simulink model "MatLab5"  (Simulink 8.7)
settings: Solver=ode45  StartTime=0.0  StopTime=100  MaxStep=0.01  RelTol=1e-3
values from neighbouring files (symbols this model uses):
  A = [0 1  0              0 ... (first row only)    [MatLab4p.m]    (also in MatLab5p.m = [     0        1       0        0; MatLab6p.m = [     0        1       0        0; _Labs.m = [     0        1       0        0; q2.m = [0 1  0   0)
  Am = blkdiag(M,M)    [MatLab5p.m]    (also in MatLab6p.m; _Labs.m; q2.m = 1; questao2.m = 1)
  B = [0; 1/M; 0; -1/(M*L)]    [MatLab4p.m]    (also in MatLab5p.m = [ 0    0; MatLab6p.m = [ 0    0; _Labs.m = [ 0    0; q2.m = [  0)
  Bm = blkdiag(N,N)    [MatLab5p.m]    (also in MatLab6p.m; _Labs.m; q2.m = N; questao2.m = N)
  C = [1 0 0 0]    [MatLab4p.m]    (also in MatLab5p.m = [1 0 0 0; MatLab6p.m = [1 0 0 0; _Labs.m = [1 0 0 0; q2.m)
  Dsim = zeros(4,1)    [MatLab4p.m]    (also in MatLab5p.m = zeros(4,2); MatLab6p.m = zeros(4,2); _Labs.m = zeros(4,2); q2.m)
  K = place(A,B,[-2 -2.05 -2.1 -2.15])    [MatLab4p.m]    (also in MatLab5p.m = Ka(:,1:4); MatLab6p.m = Ka(:,1:4); _Labs.m = Ka(:,1:4); q2.m = Ka(:,1:4))
  Km = Ka(:,5:10)    [MatLab5p.m]    (also in MatLab6p.m; _Labs.m; q2.m = Ka(5); questao2.m = Ka(:,5:7))
  x0 = [0 0 pi/4 0]    [MatLab4p.m]    (also in MatLab5p.m = [1 0.5 1 0.1]; MatLab6p.m = [1 2 0.8 -0.3]; _Labs.m = [1 2 0.8 -0.3]; q2.m = [0 0 pi/6 0])
settings Model: Creator=hector  LastModifiedBy=ivanp_o3t94tg
settings DebuggingCC: UnderspecifiedInitializationDetection=Simplified  MergeDetectMultiDrivingBlocksExec=error  SolverPrmCheckMsg=warning
settings ConfigComp: CovSFcnEnable=off

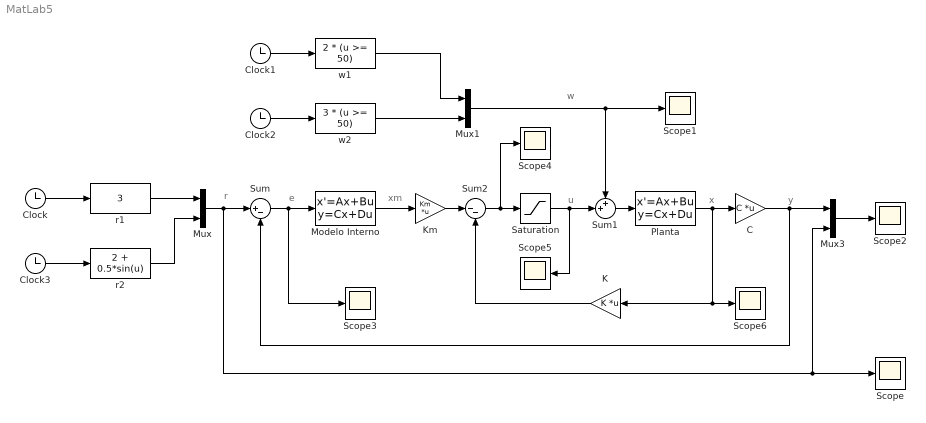
== system MatLab5 ==
  note: w
  note: u
  note: xm
  note: e
  note: r
  note: x
  note: y
  C : Gain  Gain=C  Multiplication=Matrix(K*u)
  Clock{,1..3} (4 alike) : Clock
  K : Gain  Gain=K  Multiplication=Matrix(K*u)
  Km : Gain  Gain=Km  Multiplication=Matrix(K*u)
  Modelo Interno : StateSpace  A=Am  B=Bm  C=eye(6)  D=zeros(6,2)  X0=zeros(6,1)
  Mux : Mux  Inputs=2
  Mux1 : Mux  Inputs=2
  Mux3 : Mux  Inputs=2
  Planta : StateSpace  A=A  B=B  C=eye(4)  D=Dsim  X0=x0
  Saturation : Saturate  UpperLimit=20  LowerLimit=-20
  Scope{,1..6} (7 alike) : Scope
  Sum : Sum  Inputs=|+-
  Sum1 : Sum  Inputs=++|
  Sum2 : Sum  Inputs=|--
  r1 : Fcn  Expr=3
  r2 : Fcn  Expr=2 + 0.5*sin(u)
  w1 : Fcn  Expr=2 * (u >= 50)
  w2 : Fcn  Expr=3 * (u >= 50)
  wires:
  Clock1/1 -> w1/1
  Sum/1 -> Modelo Interno/1, Scope3/1
  Sum1/1 -> Planta/1
  Clock2/1 -> w2/1
  r1/1 -> Mux/1
  Clock/1 -> r1/1
  Clock3/1 -> r2/1
  r2/1 -> Mux/2
  w1/1 -> Mux1/1
  w2/1 -> Mux1/2
  Mux1/1 -> Sum1/1, Scope1/1
  Planta/1 -> C/1, Scope6/1, K/1
  Mux3/1 -> Scope2/1
  Sum2/1 -> Saturation/1, Scope4/1
  Km/1 -> Sum2/1
  Modelo Interno/1 -> Km/1
  K/1 -> Sum2/2
  C/1 -> Mux3/1, Sum/2
  Mux/1 -> Sum/1, Scope/1, Mux3/2
  Saturation/1 -> Sum1/2, Scope5/1
